simulink model "control_law"  (R2017a)
settings: Solver=ode8  StartTime=0.0  StopTime=5  FixedStep=1e-5  RelTol=1e-3
values from neighbouring files (symbols this model uses):
  lambda = t/T    [gentrajmodel_2Drobot.m]    (also in main.m = 1; sim_model.m = 1; source_estimation.m = sestimation_info.lambda)
  nu = 2    [main.m]    (also in sim_model.m = 10; source_estimation.m = sestimation_info.nu)
  sigma = 0.5    [main.m]    (also in sim_model.m = 0.2; source_estimation.m = sestimation_info.sigma)
  T_cur = 0.1    [main.m]    (also in run_control_law.m = sestimation_info.T_cur; sim_model.m = 1)
  T_traj = 0.5    [main.m]    (also in run_control_law.m = trajectory_info.T_traj; sim_model.m = 1)
  x0 = [1; 1; 0; 1; 1; 1]    [main.m]    (also in sim_model.m = [2; 2; 0; 1; 1; 1])
undefined symbols (not defined in the file or in its folder): gaussianrnd
settings Model: Creator=brunolnetto  LastModifiedBy=brunolnetto

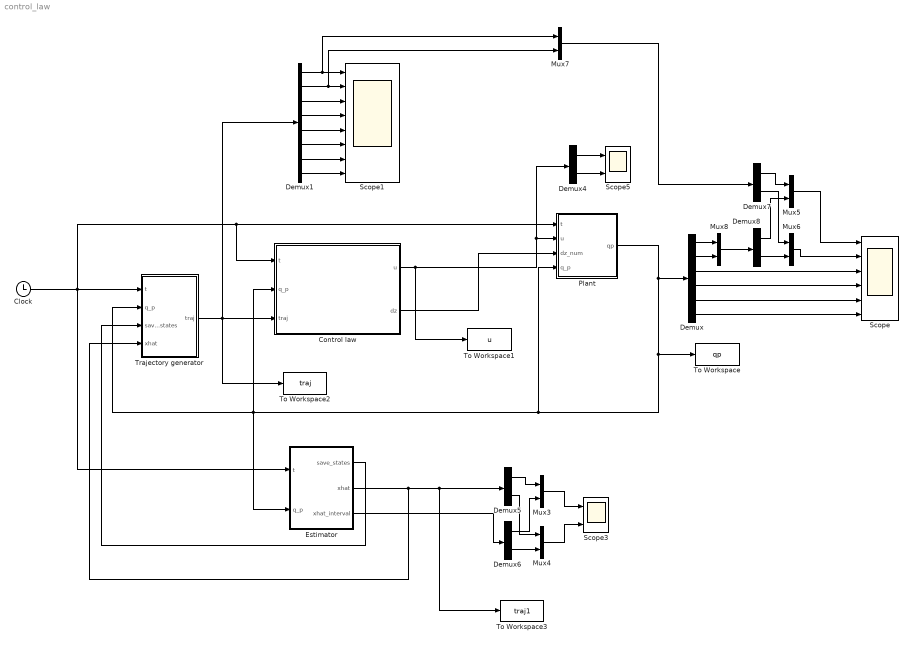
== system control_law ==
  Clock : Clock
  Control law : MATLAB Function  TreatAsAtomicUnit=on
  Demux : Demux  Outputs=6
  Demux1 : Demux  Outputs=8
  Demux{4..8} (5 alike) : Demux  Outputs=2
  Estimator : Subsystem
  Mux{3..8} (6 alike) : Mux  Inputs=2
  Plant : Subsystem
  Scope : Scope  NumInputPorts=6
  Scope1 : Scope  NumInputPorts=8
  Scope3 : Scope  NumInputPorts=2
  Scope5 : Scope  NumInputPorts=2
  To Workspace : ToWorkspace  VariableName=qp  SaveFormat=Timeseries  SampleTime=-1
  To Workspace1 : ToWorkspace  VariableName=u  SaveFormat=Timeseries  SampleTime=-1
  To Workspace2 : ToWorkspace  VariableName=traj  SaveFormat=Timeseries  SampleTime=-1
  To Workspace3 : ToWorkspace  VariableName=traj1  SaveFormat=Timeseries  SampleTime=-1
  Trajectory generator : Subsystem
  wires:
  Clock/1 -> Plant/1(t), Control law/1(t), Estimator/1(t), Trajectory generator/1(t)
  Demux/3 -> Scope/3
  Demux/4 -> Scope/4
  Demux/5 -> Scope/5
  Demux/6 -> Scope/6
  Demux4/1 -> Scope5/1
  Demux4/2 -> Scope5/2
  Demux1/3 -> Scope1/3
  Demux1/4 -> Scope1/4
  Demux1/5 -> Scope1/5
  Demux1/6 -> Scope1/6
  Demux1/7 -> Scope1/7
  Demux1/8 -> Scope1/8
  Mux3/1 -> Scope3/1
  Demux5/1 -> Mux3/1
  Demux6/1 -> Mux3/2
  Demux5/2 -> Mux4/1
  Demux6/2 -> Mux4/2
  Mux4/1 -> Scope3/2
  Mux6/1 -> Scope/2
  Demux8/2 -> Mux6/2
  Demux7/2 -> Mux6/1
  Demux8/1 -> Mux5/2
  Demux7/1 -> Mux5/1
  Mux5/1 -> Scope/1
  Demux1/2 -> Mux7/2, Scope1/2
  Demux1/1 -> Mux7/1, Scope1/1
  Mux7/1 -> Demux7/1
  Demux/1 -> Mux8/1
  Demux/2 -> Mux8/2
  Mux8/1 -> Demux8/1
  Estimator/3(xhat_interval) -> Demux6/1
  Trajectory generator/1(traj) -> To Workspace2/1, Demux1/1, Control law/3(traj)
  Estimator/1(save_states) -> Trajectory generator/3(save_states)
  Plant/1(qp) -> To Workspace/1, Trajectory generator/2(q_p), Estimator/2(q_p), Control law/2(q_p), Plant/4(q_p), Demux/1
  Control law/2(dz) -> Plant/3(dz_num)
  Control law/1(u) -> To Workspace1/1, Demux4/1, Plant/2(u)
  Estimator/2(xhat) -> To Workspace3/1, Demux5/1, Trajectory generator/4(xhat)

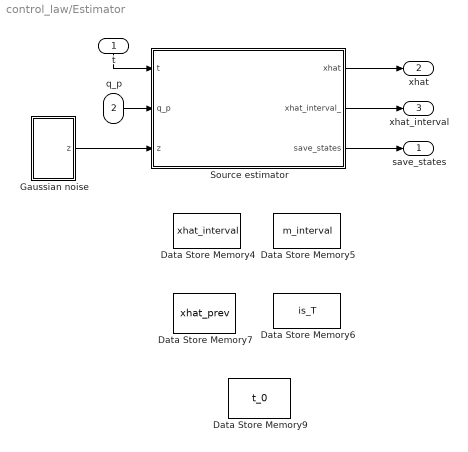
== system control_law/Estimator ==
  t : Inport
  q_p : Inport  Port=2
  Data Store Memory4 : DataStoreMemory  DataStoreName=xhat_interval  ReadBeforeWriteMsg=warning  WriteAfterWriteMsg=warning  WriteAfterReadMsg=warning  InitialValue=xhat_0  ShowAdditionalParam=off  OutDataTypeStr=double  Dimensions=[2, 1]
  Data Store Memory5 : DataStoreMemory  DataStoreName=m_interval  ReadBeforeWriteMsg=warning  WriteAfterWriteMsg=warning  WriteAfterReadMsg=warning  ShowAdditionalParam=off  OutDataTypeStr=double
  Data Store Memory6 : DataStoreMemory  DataStoreName=is_T  ReadBeforeWriteMsg=warning  WriteAfterWriteMsg=warning  WriteAfterReadMsg=warning  InitialValue=false  ShowAdditionalParam=off  OutDataTypeStr=boolean
  Data Store Memory7 : DataStoreMemory  DataStoreName=xhat_prev  ReadBeforeWriteMsg=warning  WriteAfterWriteMsg=warning  WriteAfterReadMsg=warning  InitialValue=xhat_0  ShowAdditionalParam=off  OutDataTypeStr=double
  Data Store Memory9 : DataStoreMemory  DataStoreName=t_0  ReadBeforeWriteMsg=warning  WriteAfterWriteMsg=warning  WriteAfterReadMsg=warning  ShowAdditionalParam=off  OutDataTypeStr=double
  Gaussian noise : Subsystem
  Source estimator : MATLAB Function  TreatAsAtomicUnit=on
  save_states : Outport
  xhat : Outport  Port=2
  xhat_interval : Outport  Port=3
  wires:
  t/1 -> Source estimator/1(t)
  Source estimator/2(xhat_interval_) -> xhat_interval/1
  q_p/1 -> Source estimator/2(q_p)
  Source estimator/3(save_states) -> save_states/1
  Source estimator/1(xhat) -> xhat/1
  Gaussian noise/1(z) -> Source estimator/3(z)

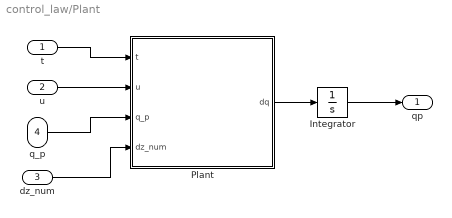
== system control_law/Plant ==
  t : Inport
  u : Inport  Port=2
  dz_num : Inport  Port=3
  q_p : Inport  Port=4
  Integrator : Integrator  InitialCondition=x0
  Plant : MATLAB Function  TreatAsAtomicUnit=on
  qp : Outport
  wires:
  t/1 -> Plant/1(t)
  q_p/1 -> Plant/3(q_p)
  u/1 -> Plant/2(u)
  Plant/1(dq) -> Integrator/1
  Integrator/1 -> qp/1
  dz_num/1 -> Plant/4(dz_num)

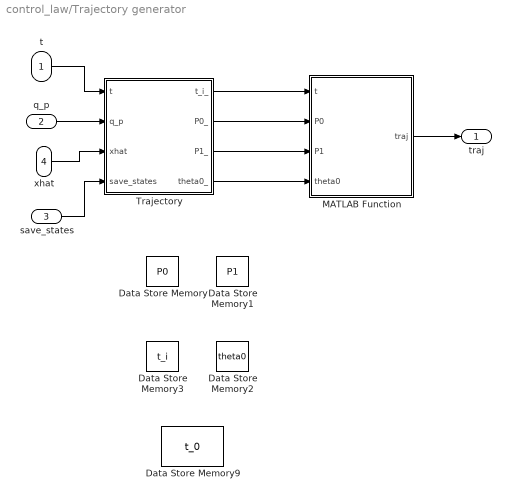
== system control_law/Trajectory generator ==
  t : Inport
  q_p : Inport  Port=2
  save_states : Inport  Port=3
  xhat : Inport  Port=4
  Data Store Memory : DataStoreMemory  DataStoreName=P0  ReadBeforeWriteMsg=warning  WriteAfterWriteMsg=warning  WriteAfterReadMsg=warning  InitialValue=x0(1:2)  ShowAdditionalParam=off  OutDataTypeStr=double  Dimensions=[2, 1]
  Data Store Memory1 : DataStoreMemory  DataStoreName=P1  ReadBeforeWriteMsg=warning  WriteAfterWriteMsg=warning  WriteAfterReadMsg=warning  InitialValue=xhat_0  ShowAdditionalParam=off  OutDataTypeStr=double
  Data Store Memory2 : DataStoreMemory  DataStoreName=theta0  ReadBeforeWriteMsg=warning  WriteAfterWriteMsg=warning  WriteAfterReadMsg=warning  InitialValue=x0(3)  ShowAdditionalParam=off  OutDataTypeStr=double
  Data Store Memory3 : DataStoreMemory  DataStoreName=t_i  ReadBeforeWriteMsg=warning  WriteAfterWriteMsg=warning  WriteAfterReadMsg=warning  ShowAdditionalParam=off  OutDataTypeStr=double
  Data Store Memory9 : DataStoreMemory  DataStoreName=t_0  ReadBeforeWriteMsg=warning  WriteAfterWriteMsg=warning  WriteAfterReadMsg=warning  ShowAdditionalParam=off  OutDataTypeStr=double
  MATLAB Function : MATLAB Function  TreatAsAtomicUnit=on
  Trajectory : MATLAB Function  TreatAsAtomicUnit=on
  traj : Outport
  wires:
  Trajectory/1(t_i_) -> MATLAB Function/1(t)
  Trajectory/4(theta0_) -> MATLAB Function/4(theta0)
  Trajectory/2(P0_) -> MATLAB Function/2(P0)
  q_p/1 -> Trajectory/2(q_p)
  MATLAB Function/1(traj) -> traj/1
  t/1 -> Trajectory/1(t)
  save_states/1 -> Trajectory/4(save_states)
  Trajectory/3(P1_) -> MATLAB Function/3(P1)
  xhat/1 -> Trajectory/3(xhat)

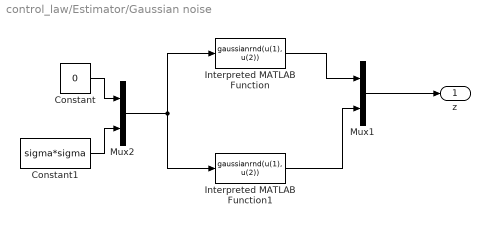
== system control_law/Estimator/Gaussian noise ==
  Constant : Constant  Value=0
  Constant1 : Constant  Value=sigma*sigma
  Interpreted MATLAB Function : MATLABFcn  MATLABFcn=gaussianrnd(u(1), u(2))  OutputSignalType=real
  Interpreted MATLAB Function1 : MATLABFcn  MATLABFcn=gaussianrnd(u(1), u(2))  OutputSignalType=real
  Mux1 : Mux  Inputs=2
  Mux2 : Mux  Inputs=2
  z : Outport
  wires:
  Interpreted MATLAB Function1/1 -> Mux1/2
  Interpreted MATLAB Function/1 -> Mux1/1
  Mux2/1 -> Interpreted MATLAB Function/1, Interpreted MATLAB Function1/1
  Constant/1 -> Mux2/1
  Mux1/1 -> z/1
  Constant1/1 -> Mux2/2

== matlab function control_law/Plant/Plant ==
  data: t input; u input; dq output; q_p input; dz_num input
function dq = plant(t, u, q_p, dz_num)
    u_1 = u(1);
    u_2 = u(2);
    
    x_1 = q_p(1);
    x_2 = q_p(2);
    x_3 = q_p(3);
    x_4 = q_p(4);
    x_5 = q_p(5);
    
    dq = [x_4.*cos(x_3);...
          x_4.*sin(x_3);...
          x_5;...
          u_1.*50 + u_2.*50;
          u_1.*8000 - u_2.*8000;
          dz_num];
end

== matlab function control_law/Control law ==
  data: t input; u output; q_p input; traj input; dz output; T_cur parameter; T_traj parameter
function [u, dz] = run_control_law(t, q_p, traj, T_cur, T_traj)   
    if(T_traj < T_cur)
        error('Trajectory plan time span must be greater than curiosity time');
    end
    
    x_1 = q_p(1);
    x_2 = q_p(2);
    x_3 = q_p(3);
    x_4 = q_p(4);
    x_5 = q_p(5);
    x_6 = q_p(6);

    x_pos_ref = traj(1);
    y_pos_ref = traj(2);
    
    xp_ref = traj(3);
    yp_ref = traj(4);
    
    xpp_ref = traj(5);
    ypp_ref = traj(6);
    
    xppp_ref = traj(7);
    yppp_ref = traj(8);
    
    % Control law
    t2 = cos(x_3);
    t3 = sin(x_3);
    t4 = x_6.*(1.0./1.0e2);
    t5 = 1.0./x_4;
    t6 = x_4.*x_5.*1.2e2;
    t7 = x_5.*x_6.*2.0;
    t8 = t2.*x_2.*6.4e4;
    t9 = t2.*y_pos_ref.*-6.4e4;
    t10 = t2.*yp_ref.*-4.8e3;
    t11 = t2.*ypp_ref.*-1.2e2;
    t12 = t3.*x_1.*-6.4e4;
    t13 = t3.*x_pos_ref.*6.4e4;
    t14 = t3.*xp_ref.*4.8e3;
    t15 = t3.*xpp_ref.*1.2e2;
    t16 = t3.*xppp_ref;
    t17 = t6+t7+t8+t9+t10+t11+t12+t13+t14+t15+t16-t2.*yppp_ref;

    u = [t4-t5.*t17.*6.25e-5;
         t4+t5.*t17.*6.25e-5];
    
    % Compensator law
    t2 = cos(x_3);
    t3 = sin(x_3);
    
    dz = x_4.*-4.8e3 - x_6.*1.2e2 - t2.*x_1.*6.4e4 - ... 
         t3.*x_2.*6.4e4 + t2.*x_pos_ref.*6.4e4 + ...
         t2.*xp_ref.*4.8e3 + t2.*xpp_ref.*1.2e2+t2.*xppp_ref + ...
         t3.*y_pos_ref.*6.4e4 + t3.*yp_ref.*4.8e3 + ...
         t3.*ypp_ref.*1.2e2+t3.*yppp_ref+x_4.*x_5.^2;
end

== matlab function control_law/Estimator/Source estimator ==
  data: t input; xhat output; xhat_interval_ output; q_p input; z input; save_states output; nu parameter; lambda parameter; T_cur parameter; xhat_interval data_store_memory; m_interval data_store_memory; xhat_prev data_store_memory; is_T data_store_memory; t_0 data_store_memory
function [xhat, xhat_interval_, save_states] = source_estimation(t, q_p, z, nu, lambda, T_cur)
    global t_0 xhat_prev m_interval xhat_interval is_T;
    
    accel_fun = @(m_1, x_1, ...
                  delta_xhat_1) non_accel(m_1, x_1, delta_xhat_1);
    oracle = @(x) x(1)^2 + x(2)^2;
    
    xhat = xhat_prev;
    save_states = is_T;
    
    % Update source estimation window
    if((t - t_0 >= T_cur)||(t == 0))
        % Quick hack: Avoid multiple reads of runge-kutta algorithm
        is_T = true;
        if(is_T)
            t_0 = t;
            
            xhat = xhat_interval + z;
            xhat_prev = xhat;
            
            % TAKE NOTE: zero xs_curr to reduce number of operations and storage
            x_curr = q_p(1:2);
            
            save_states = is_T;
            is_T = false;
        end
    end
    
    x_curr = q_p(1:2, 1);
    e_i = exp(-nu*oracle(x_curr));
    
    xhat_interval = (m_interval*xhat_interval + x_curr*e_i)/(m_interval + e_i);
    m_interval = m_interval + e_i;
    
    xhat_interval_ = xhat_interval;
end

== matlab function control_law/Trajectory generator/Trajectory ==
  data: t_i_ output; P0_ output; P1_ output; theta0_ output; t input; q_p input; xhat input; save_states input; t_0 data_store_memory; P0 data_store_memory; P1 data_store_memory; theta0 data_store_memory
function [t_i_, P0_, P1_, theta0_] = trajectory(t, q_p, xhat, save_states)
    global P0 P1 t_0 theta0;

    if(save_states)
        t_0 = t;
        
        P0 = q_p(1:2);
        P1 = xhat;
        
        theta0 = q_p(3);
        
        t_i = t - t_0;
    end
    
    P0_ = P0;
    P1_ = P1;
    theta0_ = theta0;
    t_i_ = t - t_0;
end

== matlab function control_law/Trajectory generator/MATLAB Function ==
  data: t input; traj output; P0 input; P1 input; theta0 input; T_traj parameter
function traj = line_traj(t, P0, P1, theta0, T_traj)
    traj = [P0 + (t/T_traj)*(P1 - P0); ...
            (P1 - P0)/T_traj; ...
            zeros(size(P0)); ...
            zeros(size(P0))];
end
